simulink model "stugverter_hw"  (R2026a)
settings: Solver=VariableStepAuto  StopTime=10
undefined symbols (not defined in the file): foc, FOC_20kHz, g_duty_u, g_duty_v, g_duty_w, g_foc_exec_time_us, g_foc_isr_counter
libraries: xcpprotocollib x2
settings Model: Creator=probst  LastModifiedBy=probst

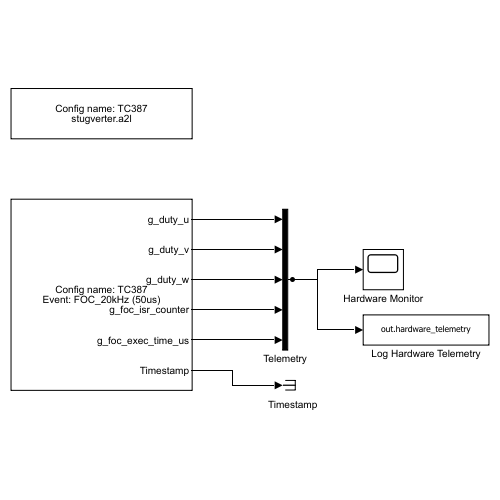
[thumbnail: Simulink's stored preview of the top-level diagram]
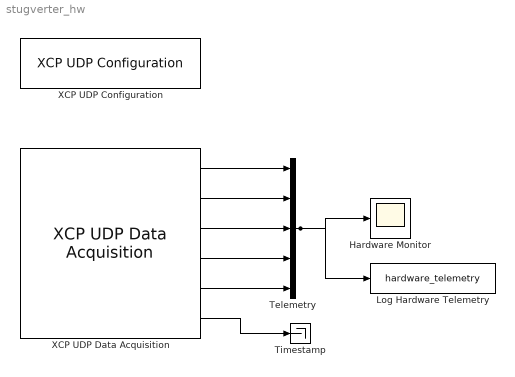
== system stugverter_hw ==
  Hardware Monitor : Scope
  Log Hardware Telemetry : ToWorkspace  VariableName=hardware_telemetry  SaveFormat=Structure With Time  SampleTime=-1
  Telemetry : Mux  Inputs=5
  Timestamp : Terminator
  XCP UDP Configuration : xcpprotocollib/UDP/XCP UDP Configuration  Priority=-100  SlaveName=TC387  SlaveID=1  A2LFile=C:\Users\probst\Desktop\stugverter\firmware\stugverter.a2l  EnableSecurity=off  ConnectMode=off  EnableStatus=off  SampleTime=foc.Ts  HeaderErrDet=on  CTRScheme=One counter for all CTOs and DTOs  LocalAddress=192.168.0.100  LocalPort=auto  DAQTimeout=Inf
      settings: LibrarySourceBlock=vntxcplib/UDP/XCP UDP Configuration
  XCP UDP Data Acquisition : xcpprotocollib/UDP/XCP UDP Data Acquisition  SlaveName=TC387  A2LFile=C:\Users\probst\Desktop\stugverter\firmware\stugverter.a2l  EventName=FOC_20kHz (50us)  SelectedMeasurements=g_duty_u;g_duty_v;g_duty_w;g_foc_isr_counter;g_foc_exec_time_us  DAQPriority=0  SampleTime=foc.Ts  EnableTimestamp=on  InputOrOutputDatatype=Raw values as double (no Compu method conversion)
      settings: LibrarySourceBlock=vntxcplib/UDP/XCP UDP Data Acquisition
  wires:
  XCP UDP Data Acquisition/1 -> Telemetry/1
  XCP UDP Data Acquisition/2 -> Telemetry/2
  XCP UDP Data Acquisition/3 -> Telemetry/3
  XCP UDP Data Acquisition/4 -> Telemetry/4
  XCP UDP Data Acquisition/5 -> Telemetry/5
  Telemetry/1 -> Hardware Monitor/1, Log Hardware Telemetry/1
  XCP UDP Data Acquisition/6 -> Timestamp/1
